simulink model "direct_forms"  (R2024b)
settings: Solver=VariableStepAuto  StartTime=0.0  StopTime=10.0  RelTol=1e-3
values from neighbouring files (symbols this model uses):
  fs = 44100    [ASL4_Bilinear.m]    (also in asl4_bilinear.m)
undefined symbols (not defined in the file or in its folder): a_1, a_2, b_0, b_1, b_2
libraries: dspsrcs4 x3
settings Model: Creator=korvo  LastModifiedBy=korvo

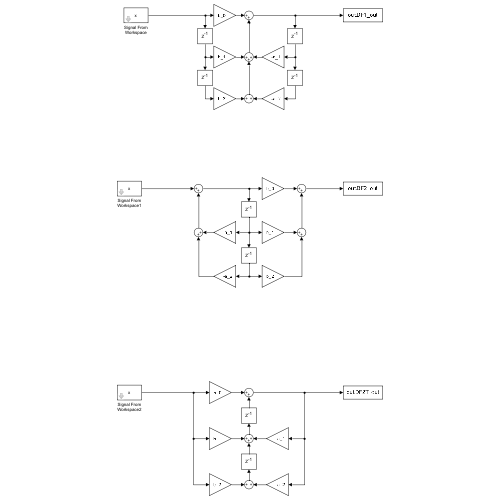
[thumbnail: Simulink's stored preview of the top-level diagram]
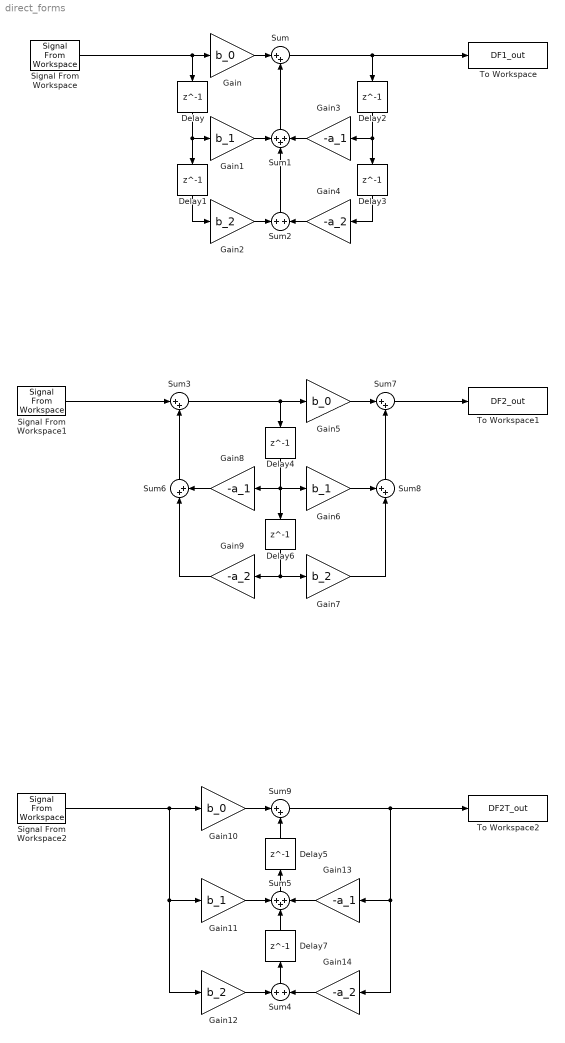
== system direct_forms ==
  Delay{,1..7} (8 alike) : Delay  DelayLength=1
  Gain : Gain  Gain=b_0
  Gain1 : Gain  Gain=b_1
  Gain10 : Gain  Gain=b_0
  Gain11 : Gain  Gain=b_1
  Gain12 : Gain  Gain=b_2
  Gain13 : Gain  Gain=-a_1
  Gain14 : Gain  Gain=-a_2
  Gain2 : Gain  Gain=b_2
  Gain3 : Gain  Gain=-a_1
  Gain4 : Gain  Gain=-a_2
  Gain5 : Gain  Gain=b_0
  Gain6 : Gain  Gain=b_1
  Gain7 : Gain  Gain=b_2
  Gain8 : Gain  Gain=-a_1
  Gain9 : Gain  Gain=-a_2
  Signal From Workspace : dspsrcs4/Signal From Workspace  X=x  Ts=1/fs  nsamps=1  OutputAfterFinalValue=Setting to zero  ignoreOrWarnInputAndFrameLengths=off  OutputFrames=off
  Signal From Workspace1 : dspsrcs4/Signal From Workspace  X=x  Ts=1/fs  nsamps=1  OutputAfterFinalValue=Setting to zero  ignoreOrWarnInputAndFrameLengths=off  OutputFrames=off
  Signal From Workspace2 : dspsrcs4/Signal From Workspace  X=x  Ts=1/fs  nsamps=1  OutputAfterFinalValue=Setting to zero  ignoreOrWarnInputAndFrameLengths=off  OutputFrames=off
  Sum{,3,6..7,9} (5 alike) : Sum  Inputs=|++
  Sum1 : Sum  Inputs=+++
  Sum2 : Sum  Inputs=+|+
  Sum4 : Sum  Inputs=+|+
  Sum5 : Sum  Inputs=+++
  Sum8 : Sum  Inputs=++|
  To Workspace : ToWorkspace  VariableName=DF1_out  SampleTime=-1
      settings: Save2DSignal=2-D array (concatenate along first dimension)
  To Workspace1 : ToWorkspace  VariableName=DF2_out  SampleTime=-1
      settings: Save2DSignal=2-D array (concatenate along first dimension)
  To Workspace2 : ToWorkspace  VariableName=DF2T_out  SampleTime=-1
      settings: Save2DSignal=2-D array (concatenate along first dimension)
  wires:
  Signal From Workspace/1 -> Delay/1, Gain/1
  Delay/1 -> Gain1/1, Delay1/1
  Delay1/1 -> Gain2/1
  Gain/1 -> Sum/1
  Gain1/1 -> Sum1/1
  Sum1/1 -> Sum/2
  Gain2/1 -> Sum2/1
  Gain4/1 -> Sum2/2
  Sum2/1 -> Sum1/2
  Gain3/1 -> Sum1/3
  Delay2/1 -> Delay3/1, Gain3/1
  Sum/1 -> To Workspace/1, Delay2/1
  Delay3/1 -> Gain4/1
  Signal From Workspace1/1 -> Sum3/1
  Sum3/1 -> Delay4/1, Gain5/1
  Gain5/1 -> Sum7/1
  Delay4/1 -> Gain8/1, Gain6/1, Delay6/1
  Gain6/1 -> Sum8/1
  Sum8/1 -> Sum7/2
  Sum7/1 -> To Workspace1/1
  Gain7/1 -> Sum8/2
  Delay6/1 -> Gain7/1, Gain9/1
  Gain8/1 -> Sum6/2
  Sum6/1 -> Sum3/2
  Gain9/1 -> Sum6/1
  Signal From Workspace2/1 -> Gain10/1, Gain12/1, Gain11/1
  Gain10/1 -> Sum9/1
  Delay5/1 -> Sum9/2
  Sum5/1 -> Delay5/1
  Gain11/1 -> Sum5/1
  Delay7/1 -> Sum5/2
  Sum4/1 -> Delay7/1
  Gain12/1 -> Sum4/1
  Gain13/1 -> Sum5/3
  Gain14/1 -> Sum4/2
  Sum9/1 -> Gain14/1, Gain13/1, To Workspace2/1
